simulink model "testableCase2"  (Simulink 8.5)
settings: Solver=FixedStepDiscrete  SolverMode=SingleTasking  StartTime=0.0  StopTime=7000  FixedStep=1  RelTol=1e-3
libraries: SimpleModeling x15
settings Model: Creator=iris  LastModifiedBy=mlab  PauseTimes=2150  SnapshotBufferSize=20  CovSFcnEnable=off
settings DataIOCC: ExternalInput=InpSignal  LimitDataPoints=off  SaveOutput=off  SignalLogging=off  SaveTime=off
settings OptimizationCC: BlockReduction=off  ConditionallyExecuteInputs=off  InlineParams=on
settings DebuggingCC: AlgebraicLoopMsg=error  SingleTaskRateTransMsg=error  FcnCallInpInsideContextMsg=UseLocalSettings
settings HardwareCC: ProdHWDeviceType=ASIC/FPGA->ASIC/FPGA  ProdEqTarget=off

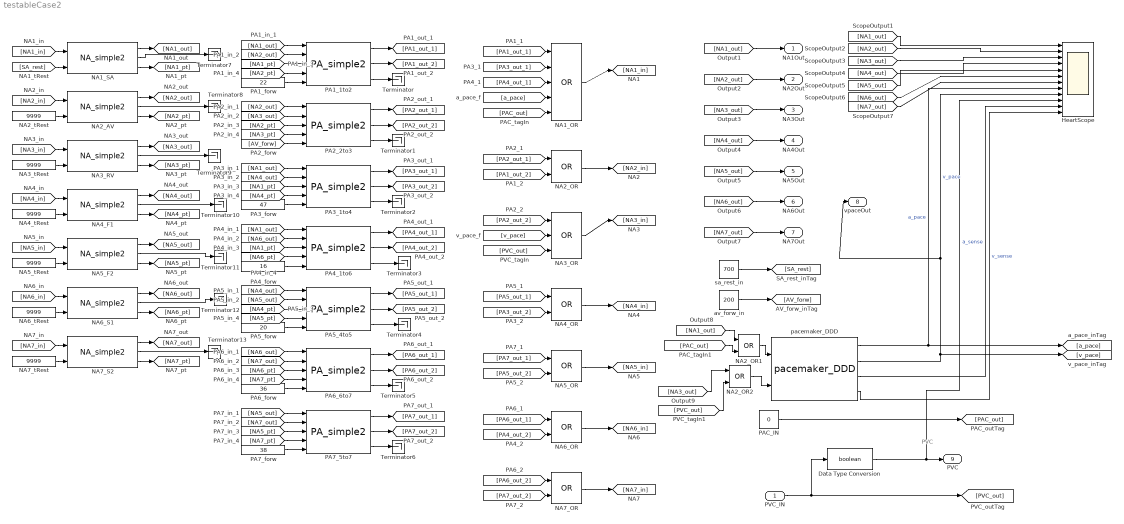
== system testableCase2 ==
  note: PVC
  PVC_IN : Inport  OutDataTypeStr=double
  Data Type Conversion : DataTypeConversion  OutDataTypeStr=boolean
  HeartScope : Scope  NumInputPorts=12
      settings: TimeRange=1500  YMin=0~0~0~0~0~0~0~-1~-1~0~-5~-5  YMax=1~1~1~1~1~1~1~1~1~1~5~5  SaveName=scopedata
  NA1_OR : Logic  Operator=OR  Inputs=5  AllPortsSameDT=off  OutDataTypeStr=boolean
  NA1_SA : SimpleModeling/NA_simple2  TERP_s_m=200  TERP_defs_m=200  TRRP_s_m=100  TRRP_def_m=100  Trest_s_m=300  Terp_min_m=200  Terp_max_m=200
  NA2_AV : SimpleModeling/NA_simple2  TERP_s_m=200  TERP_defs_m=200  TRRP_s_m=100  TRRP_def_m=100  Trest_s_m=9999  Terp_min_m=200  Terp_max_m=200
  NA2_OR : Logic  Operator=OR  AllPortsSameDT=off  OutDataTypeStr=boolean
  NA2_OR1 : Logic  Operator=OR  AllPortsSameDT=off  OutDataTypeStr=boolean
  NA2_OR2 : Logic  Operator=OR  AllPortsSameDT=off  OutDataTypeStr=boolean
  NA2_tRest : Constant  Value=9999  OutDataTypeStr=uint16
  NA3_OR : Logic  Operator=OR  Inputs=3  AllPortsSameDT=off  OutDataTypeStr=boolean
  NA3_RV : SimpleModeling/NA_simple2  TERP_s_m=250  TERP_defs_m=250  TRRP_s_m=100  TRRP_def_m=100  Trest_s_m=9999  Terp_min_m=250  Terp_max_m=250
  NA3_tRest : Constant  Value=9999  OutDataTypeStr=uint16
  NA4_F1 : SimpleModeling/NA_simple2  TERP_s_m=250  TERP_defs_m=250  TRRP_s_m=100  TRRP_def_m=100  Trest_s_m=9999  Terp_min_m=250  Terp_max_m=250
  NA4_OR : Logic  Operator=OR  AllPortsSameDT=off  OutDataTypeStr=boolean
  NA4_tRest : Constant  Value=9999  OutDataTypeStr=uint16
  NA5_F2 : SimpleModeling/NA_simple2  TERP_s_m=250  TERP_defs_m=250  TRRP_s_m=100  TRRP_def_m=100  Trest_s_m=9999  Terp_min_m=250  Terp_max_m=250
  NA5_OR : Logic  Operator=OR  AllPortsSameDT=off  OutDataTypeStr=boolean
  NA5_tRest : Constant  Value=9999  OutDataTypeStr=uint16
  NA6_OR : Logic  Operator=OR  AllPortsSameDT=off  OutDataTypeStr=boolean
  NA6_S1 : SimpleModeling/NA_simple2  TERP_s_m=150  TERP_defs_m=150  TRRP_s_m=100  TRRP_def_m=100  Trest_s_m=9999  Terp_min_m=150  Terp_max_m=150
  NA6_tRest : Constant  Value=9999  OutDataTypeStr=uint16
  NA7_OR : Logic  Operator=OR  AllPortsSameDT=off  OutDataTypeStr=boolean
  NA7_S2 : SimpleModeling/NA_simple2  TERP_s_m=150  TERP_defs_m=150  TRRP_s_m=100  TRRP_def_m=100  Trest_s_m=9999  Terp_min_m=150  Terp_max_m=150
  NA7_tRest : Constant  Value=9999  OutDataTypeStr=uint16
  PA1_1to2 : SimpleModeling/PA_simple2  min_path_par_m=10  bck_param_m=132
  PA1_forw : Constant  Value=22  OutDataTypeStr=uint16
  PA2_2to3 : SimpleModeling/PA_simple2  min_path_par_m=90  bck_param_m=144
  PA3_1to4 : SimpleModeling/PA_simple2  min_path_par_m=10  bck_param_m=32767
  PA3_forw : Constant  Value=47  OutDataTypeStr=uint16
  PA4_1to6 : SimpleModeling/PA_simple2  min_path_par_m=80  bck_param_m=16
  PA4_forw : Constant  Value=16  OutDataTypeStr=uint16
  PA5_4to5 : SimpleModeling/PA_simple2  min_path_par_m=50  bck_param_m=20
  PA5_forw : Constant  Value=20  OutDataTypeStr=uint16
  PA6_6to7 : SimpleModeling/PA_simple2  min_path_par_m=100  bck_param_m=36
  PA6_forw : Constant  Value=36  OutDataTypeStr=uint16
  PA7_5to7 : SimpleModeling/PA_simple2  min_path_par_m=50  bck_param_m=38
  PA7_forw : Constant  Value=38  OutDataTypeStr=uint16
  PAC_IN : Constant  Value=0
  Terminator{,1..13} (14 alike) : Terminator
  av_forw_in : Constant  Value=200  OutDataTypeStr=uint16
  pacemaker_DDD : SimpleModeling/pacemaker_DDD  LRI_def=1000  AVI_def=150  ARP_def=150  VRP_def=200  URI_def=400
  sa_rest_in : Constant  Value=700  OutDataTypeStr=uint16
  NA1Out : Outport
  NA2Out : Outport  Port=2
  NA3Out : Outport  Port=3
  NA4Out : Outport  Port=4
  NA5Out : Outport  Port=5
  NA6Out : Outport  Port=6
  NA7Out : Outport  Port=7
  vpaceOut : Outport  Port=8
  PVC : Outport  Port=9
  wires:
  NA1_SA/1 -> [NA1_out]
  NA1_SA/3 -> [NA1_pt]
  [NA1_in] -> NA1_SA/1
  [SA_rest] -> NA1_SA/2
  NA1_OR/1 -> [NA1_in]
  [PA1_out_1] -> NA1_OR/1
  [PA3_out_1] -> NA1_OR/2
  [PA4_out_1] -> NA1_OR/3
  [a_pace] -> NA1_OR/4
  [PAC_out] -> NA1_OR/5
  NA2_AV/1 -> [NA2_out]
  NA2_AV/3 -> [NA2_pt]
  [NA2_in] -> NA2_AV/1
  NA2_tRest/1 -> NA2_AV/2
  NA2_OR/1 -> [NA2_in]
  [PA2_out_1] -> NA2_OR/1
  [PA1_out_2] -> NA2_OR/2
  NA3_RV/1 -> [NA3_out]
  NA3_RV/3 -> [NA3_pt]
  [NA3_in] -> NA3_RV/1
  NA3_tRest/1 -> NA3_RV/2
  NA3_OR/1 -> [NA3_in]
  [PA2_out_2] -> NA3_OR/1
  [v_pace] -> NA3_OR/2
  [PVC_out] -> NA3_OR/3
  NA4_F1/1 -> [NA4_out]
  NA4_F1/3 -> [NA4_pt]
  [NA4_in] -> NA4_F1/1
  NA4_tRest/1 -> NA4_F1/2
  NA4_OR/1 -> [NA4_in]
  [PA5_out_1] -> NA4_OR/1
  [PA3_out_2] -> NA4_OR/2
  NA5_F2/1 -> [NA5_out]
  NA5_F2/3 -> [NA5_pt]
  [NA5_in] -> NA5_F2/1
  NA5_tRest/1 -> NA5_F2/2
  NA5_OR/1 -> [NA5_in]
  [PA7_out_1] -> NA5_OR/1
  [PA5_out_2] -> NA5_OR/2
  NA6_S1/1 -> [NA6_out]
  NA6_S1/3 -> [NA6_pt]
  [NA6_in] -> NA6_S1/1
  NA6_tRest/1 -> NA6_S1/2
  NA6_OR/1 -> [NA6_in]
  [PA6_out_1] -> NA6_OR/1
  [PA4_out_2] -> NA6_OR/2
  NA7_S2/1 -> [NA7_out]
  NA7_S2/3 -> [NA7_pt]
  [NA7_in] -> NA7_S2/1
  NA7_tRest/1 -> NA7_S2/2
  NA7_OR/1 -> [NA7_in]
  [PA6_out_2] -> NA7_OR/1
  [PA7_out_2] -> NA7_OR/2
  PA1_1to2/1 -> [PA1_out_1]
  PA1_1to2/2 -> [PA1_out_2]
  [NA1_out] -> PA1_1to2/1
  [NA2_out] -> PA1_1to2/2
  [NA1_pt] -> PA1_1to2/3
  [NA2_pt] -> PA1_1to2/4
  PA1_forw/1 -> PA1_1to2/5
  PA2_2to3/1 -> [PA2_out_1]
  PA2_2to3/2 -> [PA2_out_2]
  [NA2_out] -> PA2_2to3/1
  [NA3_out] -> PA2_2to3/2
  [NA2_pt] -> PA2_2to3/3
  [NA3_pt] -> PA2_2to3/4
  [AV_forw] -> PA2_2to3/5
  PA3_1to4/1 -> [PA3_out_1]
  PA3_1to4/2 -> [PA3_out_2]
  [NA1_out] -> PA3_1to4/1
  [NA4_out] -> PA3_1to4/2
  [NA1_pt] -> PA3_1to4/3
  [NA4_pt] -> PA3_1to4/4
  PA3_forw/1 -> PA3_1to4/5
  PA4_1to6/1 -> [PA4_out_1]
  PA4_1to6/2 -> [PA4_out_2]
  [NA1_out] -> PA4_1to6/1
  [NA6_out] -> PA4_1to6/2
  [NA1_pt] -> PA4_1to6/3
  [NA6_pt] -> PA4_1to6/4
  PA4_forw/1 -> PA4_1to6/5
  PA5_4to5/1 -> [PA5_out_1]
  PA5_4to5/2 -> [PA5_out_2]
  [NA4_out] -> PA5_4to5/1
  [NA5_out] -> PA5_4to5/2
  [NA4_pt] -> PA5_4to5/3
  [NA5_pt] -> PA5_4to5/4
  PA5_forw/1 -> PA5_4to5/5
  PA6_6to7/1 -> [PA6_out_1]
  PA6_6to7/2 -> [PA6_out_2]
  [NA6_out] -> PA6_6to7/1
  [NA7_out] -> PA6_6to7/2
  [NA6_pt] -> PA6_6to7/3
  [NA7_pt] -> PA6_6to7/4
  PA6_forw/1 -> PA6_6to7/5
  PA7_5to7/1 -> [PA7_out_1]
  PA7_5to7/2 -> [PA7_out_2]
  [NA5_out] -> PA7_5to7/1
  [NA7_out] -> PA7_5to7/2
  [NA5_pt] -> PA7_5to7/3
  [NA7_pt] -> PA7_5to7/4
  PA7_forw/1 -> PA7_5to7/5
  [NA1_out] -> NA1Out/1
  [NA2_out] -> NA2Out/1
  [NA3_out] -> NA3Out/1
  [NA4_out] -> NA4Out/1
  [NA5_out] -> NA5Out/1
  [NA6_out] -> NA6Out/1
  [NA7_out] -> NA7Out/1
  sa_rest_in/1 -> [SA_rest]
  av_forw_in/1 -> [AV_forw]
  [NA1_out] -> HeartScope/1
  [NA2_out] -> HeartScope/2
  [NA3_out] -> HeartScope/3
  [NA4_out] -> HeartScope/4
  [NA5_out] -> HeartScope/5
  [NA6_out] -> HeartScope/6
  [NA7_out] -> HeartScope/7
  pacemaker_DDD/1 -> HeartScope/8, [a_pace]  "a_pace"
  pacemaker_DDD/2 -> vpaceOut/1, HeartScope/9, [v_pace]  "v_pace"
  [NA1_out] -> NA2_OR1/1
  [PAC_out] -> NA2_OR1/2
  NA2_OR1/1 -> pacemaker_DDD/1
  [NA3_out] -> NA2_OR2/1
  [PVC_out] -> NA2_OR2/2
  NA2_OR2/1 -> pacemaker_DDD/2
  PAC_IN/1 -> [PAC_out]
  PVC_IN/1 -> Data Type Conversion/1, [PVC_out]
  Data Type Conversion/1 -> HeartScope/10, PVC/1
  pacemaker_DDD/3 -> HeartScope/11  "a_sense"
  pacemaker_DDD/4 -> HeartScope/12  "v_sense"
  PA1_1to2/3 -> Terminator/1
  PA2_2to3/3 -> Terminator1/1
  PA3_1to4/3 -> Terminator2/1
  PA4_1to6/3 -> Terminator3/1
  PA5_4to5/3 -> Terminator4/1
  PA6_6to7/3 -> Terminator5/1
  PA7_5to7/3 -> Terminator6/1
  NA1_SA/2 -> Terminator7/1
  NA2_AV/2 -> Terminator8/1
  NA3_RV/2 -> Terminator9/1
  NA4_F1/2 -> Terminator10/1
  NA5_F2/2 -> Terminator11/1
  NA6_S1/2 -> Terminator12/1
  NA7_S2/2 -> Terminator13/1
